simulink model "ftjlk"  (R2023a)
settings: Solver=VariableStepAuto  StartTime=0.0  StopTime=2  RelTol=1e-3
model workspace (MAT data in the model file):
  Kc = Simulink.Parameter
  Kc.DataType = 'auto'
  Kc.Complexity = 'real'
  Kc.Dimensions = [0 0]
  a = Simulink.Parameter
  a.DataType = 'auto'
  a.Complexity = 'real'
  a.Dimensions = [0 0]
settings Model: Creator=1  LastModifiedBy=ASUS
settings DebuggingCC: UnconnectedInputMsg=warning  UnconnectedOutputMsg=warning  UnconnectedLineMsg=warning
settings ModelReferenceCC: EnableRefExpFcnMdlSchedulingChecks=on
settings RTWCC: DLArmComputeVersion=19.05

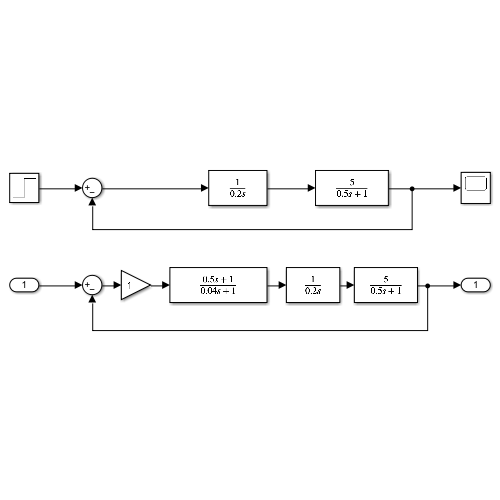
[thumbnail: Simulink's stored preview of the top-level diagram]
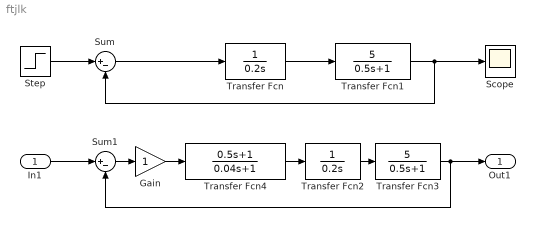
== system ftjlk ==
  In1 : Inport
  Gain : Gain
  Scope : Scope
  Step : Step  After=5  SampleTime=0
  Sum : Sum  Inputs=|+-
  Sum1 : Sum  Inputs=|+-
  Transfer Fcn : TransferFcn  Denominator=[0.2 0]
  Transfer Fcn1 : TransferFcn  Numerator=[5]  Denominator=[0.5 1]
  Transfer Fcn2 : TransferFcn  Denominator=[0.2 0]
  Transfer Fcn3 : TransferFcn  Numerator=[5]  Denominator=[0.5 1]
  Transfer Fcn4 : TransferFcn  Numerator=[0.5 1]  Denominator=[0.04 1]
  Out1 : Outport
  wires:
  Sum/1 -> Transfer Fcn/1
  Transfer Fcn/1 -> Transfer Fcn1/1
  Transfer Fcn1/1 -> Scope/1, Sum/2
  Transfer Fcn2/1 -> Transfer Fcn3/1
  Transfer Fcn3/1 -> Out1/1, Sum1/2
  Transfer Fcn4/1 -> Transfer Fcn2/1
  Sum1/1 -> Gain/1
  Gain/1 -> Transfer Fcn4/1
  In1/1 -> Sum1/1
  Step/1 -> Sum/1
